simulink model "completeWithSubSystems"  (R2020a)
settings: Solver=VariableStepAuto  StartTime=0.0  StopTime=10.0  RelTol=1e-3
libraries: simulink x2
settings Model: Creator=shrad  LastModifiedBy=shrad

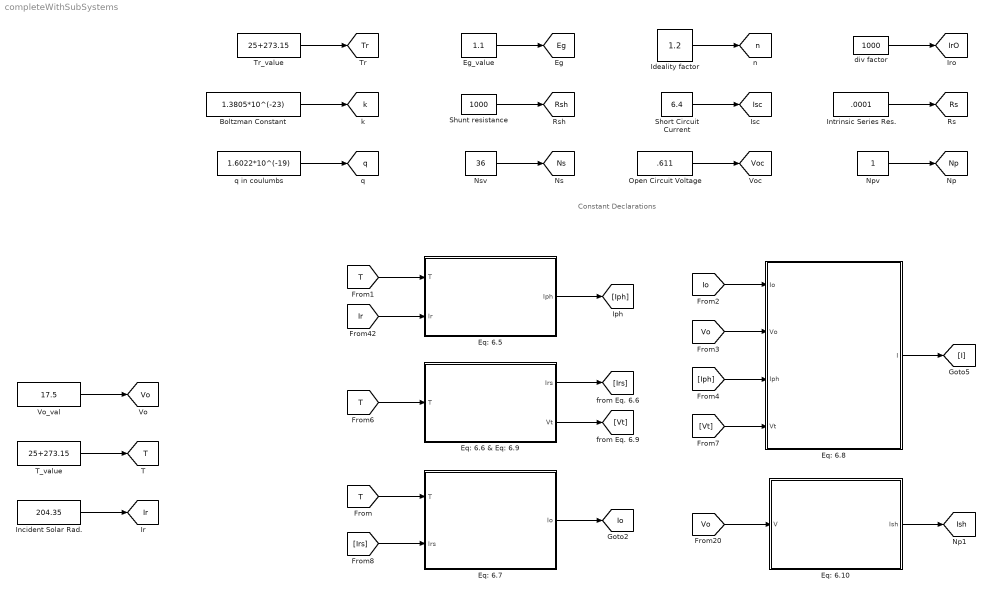
== system completeWithSubSystems ==
  note: Constant Declarations
  Boltzman Constant : Constant  Value=1.3805*10^(-23)
  Eg_value : Constant  Value=1.1
  Eq: 6.10 : Subsystem
  Eq: 6.5 : Subsystem
  Eq: 6.6 & Eq: 6.9 : Subsystem
  Eq: 6.7 : Subsystem
  Eq: 6.8 : Subsystem
  Ideality factor : Constant  Value=1.2
  Incident Solar Rad. : Constant  Value=204.35
  Intrinsic Series Res. : Constant  Value=.0001
  Npv : Constant
  Nsv : Constant  Value=36
  Open Circuit Voltage : Constant  Value=.611
  Short Circuit Current : Constant  Value=6.4
  Shunt resistance : Constant  Value=1000
  T_value : Constant  Value=25+273.15
  Tr_value : Constant  Value=25+273.15
  Vo_val : Constant  Value=17.5
  div factor : Constant  Value=1000
  q in coulumbs : Constant  Value=1.6022*10^(-19)
  tag scope: Eg=global, Io=global, Ir=global, IrO=global, Isc=global, Ish=global, Np=global, Ns=global, Rs=global, Rsh=global, T=global, Tr=global, Vo=global, Voc=global, k=global, n=global, q=global
  wires:
  Incident Solar Rad./1 -> [Ir]
  Ideality factor/1 -> [n]
  Open Circuit Voltage/1 -> [Voc]
  T_value/1 -> [T]
  q in coulumbs/1 -> [q]
  div factor/1 -> [IrO]
  Boltzman Constant/1 -> [k]
  Tr_value/1 -> [Tr]
  Shunt resistance/1 -> [Rsh]
  Short Circuit Current/1 -> [Isc]
  Npv/1 -> [Np]
  Nsv/1 -> [Ns]
  Intrinsic Series Res./1 -> [Rs]
  Eg_value/1 -> [Eg]
  [T] -> Eq: 6.6 & Eq: 6.9/1(T)
  [T] -> Eq: 6.7/1(T)
  Eq: 6.7/1(Io) -> [Io]
  [Vo] -> Eq: 6.10/1(V)
  Eq: 6.8/1(I) -> [I]
  [Io] -> Eq: 6.8/1(Io)
  [Iph] -> Eq: 6.8/3(Iph)
  Vo_val/1 -> [Vo]
  [T] -> Eq: 6.5/1(T)
  [Ir] -> Eq: 6.5/2(Ir)
  Eq: 6.5/1(Iph) -> [Iph]
  Eq: 6.6 & Eq: 6.9/1(Irs) -> [Irs]
  Eq: 6.6 & Eq: 6.9/2(Vt) -> [Vt]
  [Vo] -> Eq: 6.8/2(Vo)
  [Vt] -> Eq: 6.8/4(Vt)
  [Irs] -> Eq: 6.7/2(Irs)
  Eq: 6.10/1(Ish) -> [Ish]

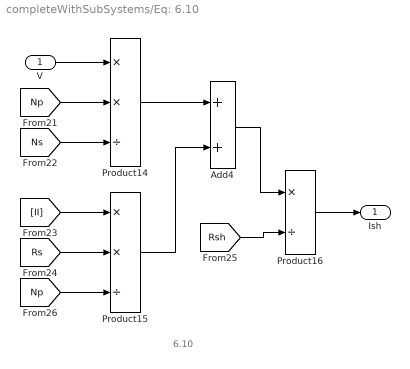
== system completeWithSubSystems/Eq: 6.10 ==
  note: 6.10
  V : Inport
  Add4 : Sum
  Product14 : Product  Inputs=**/
  Product15 : Product  Inputs=**/
  Product16 : Product  Inputs=*/
  Ish : Outport
  wires:
  Product14/1 -> Add4/1
  Product16/1 -> Ish/1
  [Np] -> Product15/3
  [Rs] -> Product15/2
  [Ns] -> Product14/3
  Add4/1 -> Product16/1
  [II] -> Product15/1
  [Rsh] -> Product16/2
  [Np] -> Product14/2
  Product15/1 -> Add4/2
  V/1 -> Product14/1

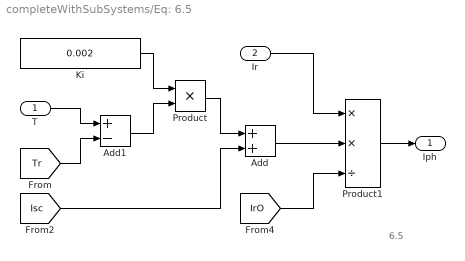
== system completeWithSubSystems/Eq: 6.5 ==
  note: 6.5
  T : Inport
  Ir : Inport  Port=2
  Add : Sum
  Add1 : Sum  Inputs=+-
  Ki : Constant  Value=0.002
  Product : Product
  Product1 : Product  Inputs=**/
  Iph : Outport
  wires:
  Product/1 -> Add/1
  Ir/1 -> Product1/1
  Add1/1 -> Product/2
  Add/1 -> Product1/2
  T/1 -> Add1/1
  Ki/1 -> Product/1
  [Tr] -> Add1/2
  [IrO] -> Product1/3
  Product1/1 -> Iph/1
  [Isc] -> Add/2

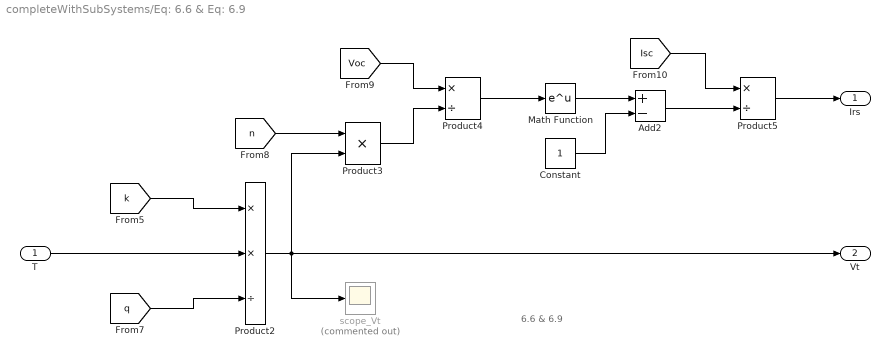
== system completeWithSubSystems/Eq: 6.6 & Eq: 6.9 ==
  note: 6.6 & 6.9
  T : Inport
  Add2 : Sum  Inputs=+-
  Constant : Constant
  Math Function : Math  SaturateOnIntegerOverflow=on
  Product2 : Product  Inputs=**/
  Product3 : Product
  Product4 : Product  Inputs=*/
  Product5 : Product  Inputs=*/
  scope_Vt : Scope  Commented=on
  Irs : Outport
  Vt : Outport  Port=2
  wires:
  Product4/1 -> Math Function/1
  [k] -> Product2/1
  [q] -> Product2/3
  [Isc] -> Product5/1
  Add2/1 -> Product5/2
  Constant/1 -> Add2/2
  [n] -> Product3/1
  Product3/1 -> Product4/2
  [Voc] -> Product4/1
  Math Function/1 -> Add2/1
  Product2/1 -> Vt/1, Product3/2, scope_Vt/1
  Product5/1 -> Irs/1
  T/1 -> Product2/2

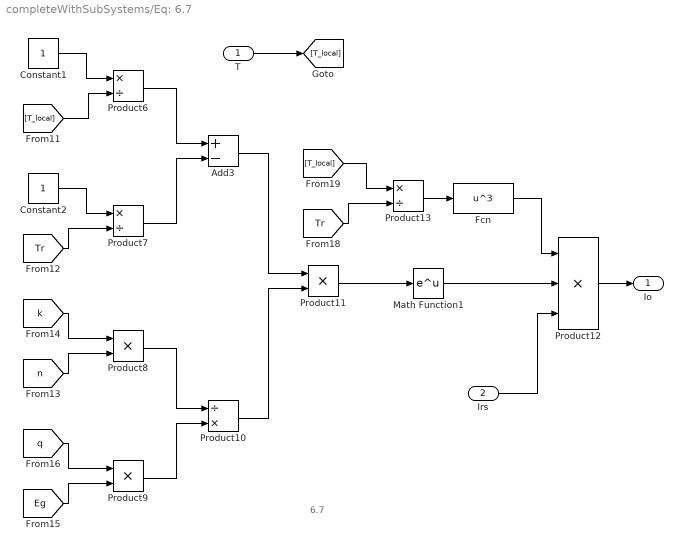
== system completeWithSubSystems/Eq: 6.7 ==
  note: 6.7
  T : Inport
  Irs : Inport  Port=2
  Add3 : Sum  Inputs=+-
  Constant1 : Constant
  Constant2 : Constant
  Fcn : Fcn  Expr=u^3
  Math Function1 : Math  SaturateOnIntegerOverflow=on
  Product10 : Product  Inputs=/*
  Product11 : Product  Inputs=**
  Product12 : Product  Inputs=***
  Product13 : Product  Inputs=*/
  Product6 : Product  Inputs=*/
  Product7 : Product  Inputs=*/
  Product8 : Product  Inputs=**
  Product9 : Product  Inputs=**
  Io : Outport
  wires:
  Math Function1/1 -> Product12/2
  [n] -> Product8/2
  Product7/1 -> Add3/2
  Constant2/1 -> Product7/1
  Product13/1 -> Fcn/1
  Fcn/1 -> Product12/1
  [T_local] -> Product13/1
  Irs/1 -> Product12/3
  [k] -> Product8/1
  Add3/1 -> Product11/1
  Product12/1 -> Io/1
  Product9/1 -> Product10/2
  Product11/1 -> Math Function1/1
  [q] -> Product9/1
  [T_local] -> Product6/2
  Constant1/1 -> Product6/1
  [Eg] -> Product9/2
  Product10/1 -> Product11/2
  [Tr] -> Product13/2
  Product8/1 -> Product10/1
  T/1 -> [T_local]
  Product6/1 -> Add3/1
  [Tr] -> Product7/2

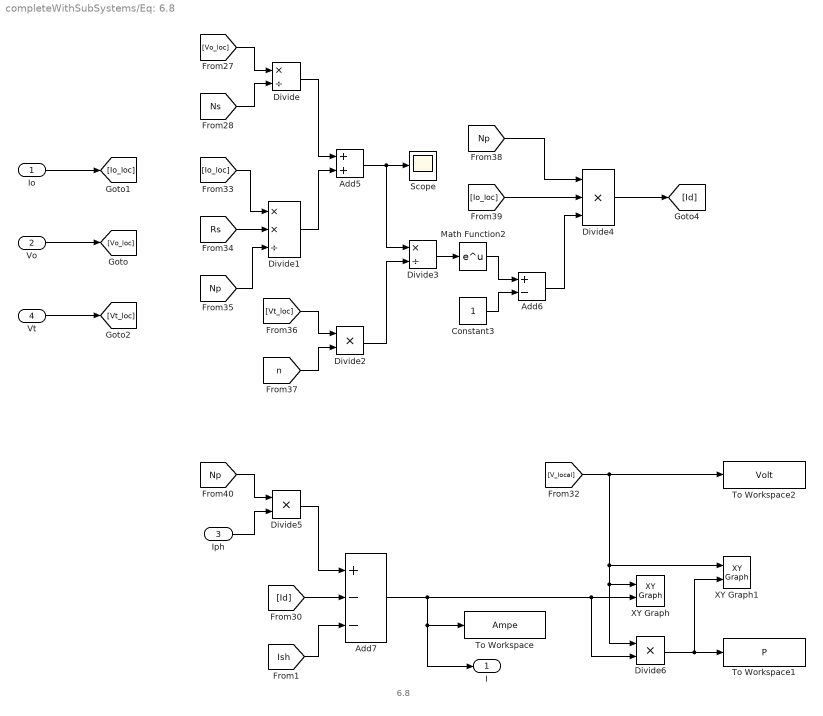
== system completeWithSubSystems/Eq: 6.8 ==
  note: 6.8
  Io : Inport
  Vo : Inport  Port=2
  Iph : Inport  Port=3
  Vt : Inport  Port=4
  Add5 : Sum
  Add6 : Sum  Inputs=+-
  Add7 : Sum  Inputs=+--
  Constant3 : Constant
  Divide : Product  Inputs=*/
  Divide1 : Product  Inputs=**/
  Divide2 : Product
  Divide3 : Product  Inputs=*/
  Divide4 : Product  Inputs=3
  Divide5 : Product
  Divide6 : Product
  Math Function2 : Math  SaturateOnIntegerOverflow=on
  Scope : Scope
  To Workspace : ToWorkspace  VariableName=Ampe  SaveFormat=Timeseries  SampleTime=-1
  To Workspace1 : ToWorkspace  VariableName=P  SaveFormat=Timeseries  SampleTime=-1
  To Workspace2 : ToWorkspace  VariableName=Volt  SaveFormat=Timeseries  SampleTime=-1
  XY Graph : simulink/Sinks/XY Graph  xmin=-1  xmax=1  ymin=-1  ymax=1  st=-1
  XY Graph1 : simulink/Sinks/XY Graph  xmin=-1  xmax=1  ymin=-1  ymax=1  st=-1
  I : Outport
  wires:
  [n] -> Divide2/2
  Divide2/1 -> Divide3/2
  Divide4/1 -> [Id]
  Add7/1 -> I/1, To Workspace/1, Divide6/2, XY Graph/2
  Divide5/1 -> Add7/1
  [Ns] -> Divide/2
  [Np] -> Divide5/1
  Divide6/1 -> To Workspace1/1, XY Graph1/2
  [Vo_loc] -> Divide/1
  Divide1/1 -> Add5/2
  Math Function2/1 -> Add6/1
  [Ish] -> Add7/3
  [Np] -> Divide4/1
  [Rs] -> Divide1/2
  Divide3/1 -> Math Function2/1
  [Np] -> Divide1/3
  Iph/1 -> Divide5/2
  Divide/1 -> Add5/1
  Add6/1 -> Divide4/3
  [Vt_loc] -> Divide2/1
  [Io_loc] -> Divide4/2
  [V_local] -> To Workspace2/1, XY Graph1/1, Divide6/1, XY Graph/1
  Add5/1 -> Scope/1, Divide3/1
  Constant3/1 -> Add6/2
  [Id] -> Add7/2
  [Io_loc] -> Divide1/1
  Io/1 -> [Io_loc]
  Vo/1 -> [Vo_loc]
  Vt/1 -> [Vt_loc]
